simulink model "UART_Debug"  (R2020b)
settings: Solver=FixedStepDiscrete  StartTime=0.0  StopTime=inf  FixedStep=0.1  RelTol=1e-3
PreLoadFcn:
  | cd(fileparts(which(bdroot)));
InitFcn:
  | set_param([bdroot,'/refIq'], 'value','0');
  | set_param([bdroot, '/cmd'], 'value', '0');
  | set_param([bdroot, '/refRPM'], 'value', '0');
libraries: mcbhostblockslib x3
PreSaveFcn:
  | cd(fileparts(which(bdroot)));
settings Model: Creator=beau_  LastModifiedBy=Administrator
settings DataIOCC: SaveOutput=off  SignalLogging=off  DSMLogging=off  SaveTime=off  ReturnWorkspaceOutputs=off

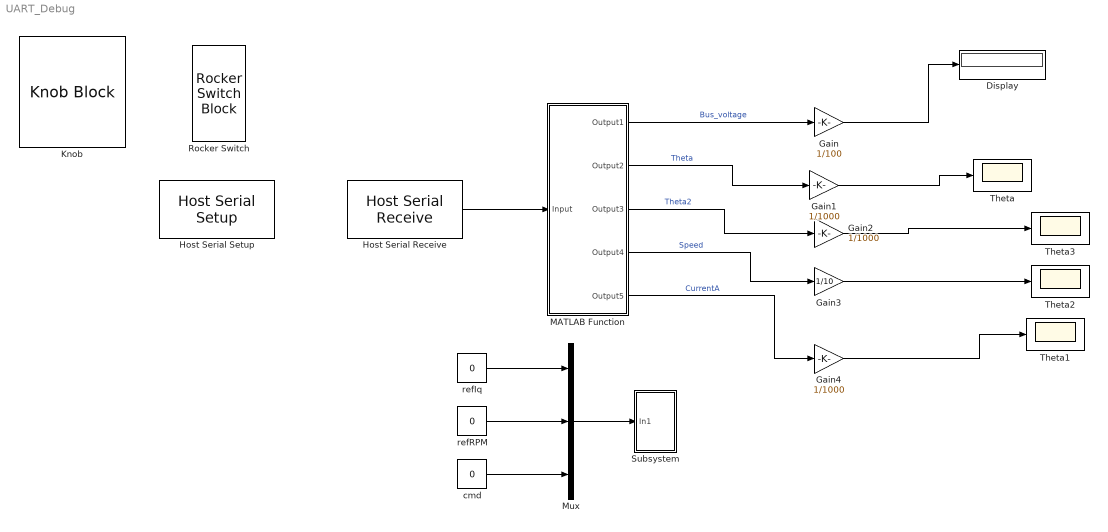
== system UART_Debug ==
  Display : Display
  Gain : Gain  Gain=1/100
  Gain1 : Gain  Gain=1/1000
  Gain2 : Gain  Gain=1/1000
  Gain3 : Gain  Gain=1/10
  Gain4 : Gain  Gain=1/1000
  Host Serial Receive : mcbhostblockslib/Host Serial Receive  serialCon=Serial 1  dataHead='AA'  dataTail='BB'  dataType=int16  dataDim=[1000,5]  initValue=0  errOption=Output custom value  errValue=0  sampleTime=0.5  outputStatus=off  blockingMode=on
      settings: SourceProductBaseCode=MT
  Host Serial Setup : mcbhostblockslib/Host Serial Setup  Priority=-99  comPortSer1='COM3'  baudRateA=750000  charLenA=8  stopBitA=1  parityA=none  timeoutA=1.0  ByteOrderA=LittleEndian  comPortSer2='Please_select_a_port'  baudRateB=115200  charLenB=8  stopBitB=1  parityB=none  timeoutB=1.0  ByteOrderB=LittleEndian  comPortSer3='Please_select_a_port'  baudRateC=115200  charLenC=8  stopBitC=1  parityC=none  timeoutC=1.0  ByteOrderC=LittleEndian  comPortSer4='Please_select_a_port'  baudRateD=115200  charLenD=8  stopBitD=1  parityD=none  timeoutD=1.0  ByteOrderD=LittleEndian
      settings: SourceProductBaseCode=MT
  Knob : KnobBlock  ScaleMin=-1600  ScaleMax=1600
  MATLAB Function : MATLAB Function  TreatAsAtomicUnit=on
  Mux : Mux  Inputs=3
  Rocker Switch : RockerSwitchBlock
      settings: Values={{'Off', 'On'}, [0 1]}
  Subsystem : Subsystem  TreatAsAtomicUnit=on  SystemSampleTime=0.2
  Theta{,1..3} (4 alike) : Scope
  cmd : Constant  Value=0
  refIq : Constant  Value=0
  refRPM : Constant  Value=0
  wires:
  Host Serial Receive/1 -> MATLAB Function/1(Input)
  refIq/1 -> Mux/1
  Mux/1 -> Subsystem/1(In1)
  refRPM/1 -> Mux/2
  cmd/1 -> Mux/3
  MATLAB Function/1(Output1) -> Gain/1  "Bus_voltage"
  MATLAB Function/2(Output2) -> Gain1/1  "Theta"
  MATLAB Function/3(Output3) -> Gain2/1  "Theta2"
  MATLAB Function/4(Output4) -> Gain3/1  "Speed"
  MATLAB Function/5(Output5) -> Gain4/1  "CurrentA"
  Gain/1 -> Display/1
  Gain4/1 -> Theta1/1
  Gain3/1 -> Theta2/1
  Gain2/1 -> Theta3/1
  Gain1/1 -> Theta/1

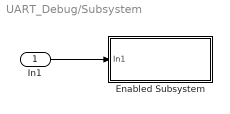
== system UART_Debug/Subsystem ==
  In1 : Inport
  Enabled Subsystem : Subsystem  TreatAsAtomicUnit=on
  wires:
  In1/1 -> Enabled Subsystem/1(In1)

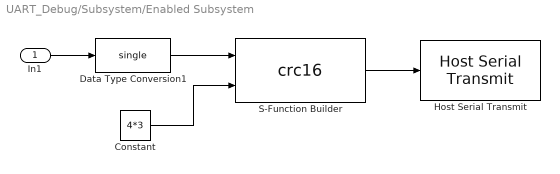
== system UART_Debug/Subsystem/Enabled Subsystem ==
  In1 : Inport
  Constant : Constant  Value=4*3  OutDataTypeStr=single  SampleTime=-1
  Data Type Conversion1 : DataTypeConversion  OutDataTypeStr=single
  Host Serial Transmit : mcbhostblockslib/Host Serial Transmit  serialCon=Serial 1  header=''  tail=''  enableBlockingMode=off
      settings: SourceProductBaseCode=MT
  S-Function Builder : S-Function  FunctionName=crc16  SFunctionModules=crc16_wrapper  SFunctionDeploymentMode=off  EnableBusSupport=off  mask(S-Function Builder){}
      mask help: Simulink:masks:SFunctionBuilder_MD
      mask init:
      | val = [[.9  0.75 0.75 1 1 .9 .9 1]',[1 1 0.75 0.75 .9 .9 1 .9]'];try , sys = get_param(gcb,'SfunBuilderFcnName');if isempty(sys), sys = get_param(gcb,'FunctionName'); end,catch, sys = get_param(gcb,'FunctionName'); end
      settings: CopyFcn=set_param(gcbh,'LinkStatus','none')  OpenFcn=sfunctionwizard(gcbh)
      mask Display:
      | plot(val(:,1),val(:,2))
      | disp(sys)
      | port_label('input',1,'ptr')
      | port_label('input',2,'len')
      | port_label('output',1,'crcOut')
  wires:
  In1/1 -> Data Type Conversion1/1
  S-Function Builder/1 -> Host Serial Transmit/1
  Data Type Conversion1/1 -> S-Function Builder/1
  Constant/1 -> S-Function Builder/2

== matlab function UART_Debug/MATLAB Function ==
  data: Input input; Output1 output; Output2 output; Output3 output; Output4 output; Output5 output
function [Output1,Output2,Output3,Output4,Output5]  = unBuf(Input)

Output1 = Input(:, 1);
Output2 = Input(:, 2);
Output3 = Input(:, 3);
Output4 = Input(:, 4);
Output5 = Input(:, 5);

end
